simulink model "POParAgRL"  (R2015a)
settings: Solver=ode45  StartTime=0.0  StopTime=3  FixedStep=0.00001  RelTol=1e-5
settings Model: Creator=user  LastModifiedBy=user
settings SolverCC: ZeroCrossAlgorithm=Adaptive
settings DebuggingCC: UnderspecifiedInitializationDetection=Classic

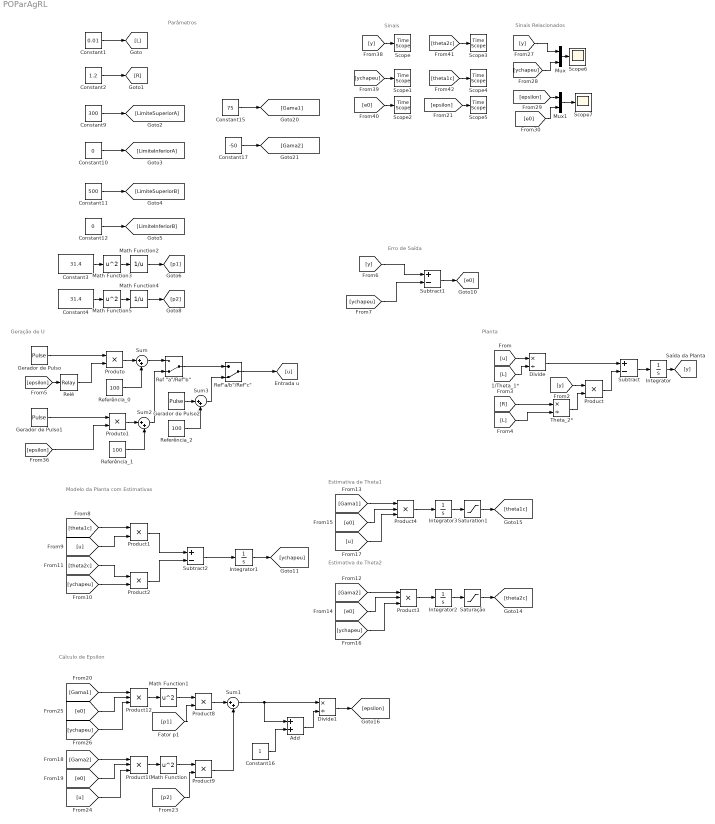
== system POParAgRL ==
  note: Modelo da Planta com Estimativas
  note: Sinais Relacionados
  note: Cálculo de Epsilon
  note: Estimativa de Theta1
  note: Estimativa de Theta2
  note: Geração de U
  note: Erro de Saída
  note: Parâmetros
  note: Sinais
  note: Planta
  Add : Sum  AccumDataTypeStr=double
  Constant1 : Constant  Value=0.01
  Constant10 : Constant  Value=0
  Constant11 : Constant  Value=500
  Constant12 : Constant  Value=0
  Constant15 : Constant  Value=75
  Constant16 : Constant
  Constant17 : Constant  Value=-50
  Constant2 : Constant  Value=1.2
  Constant3 : Constant  Value=31.4
  Constant4 : Constant  Value=31.4
  Constant9 : Constant  Value=300
  Divide : Product  Inputs=*/
  Divide1 : Product  Inputs=*/  OutDataTypeStr=double
  Gerador de Pulso : DiscretePulseGenerator  PulseType=Time based  Amplitude=100  Period=0.01  PulseWidth=50
  Gerador de Pulso1 : DiscretePulseGenerator  PulseType=Time based  Amplitude=100  Period=0.01  PulseWidth=50
  Gerador de Pulso2 : DiscretePulseGenerator  PulseType=Time based  Amplitude=100  Period=0.01  PulseWidth=50
  Integrator : Integrator
  Integrator1 : Integrator
  Integrator2 : Integrator  InitialCondition=70
  Integrator3 : Integrator  InitialCondition=80
  Math Function{,1,3,5} (4 alike) : Math  Operator=square  SaturateOnIntegerOverflow=on
  Math Function2 : Math  Operator=reciprocal  SaturateOnIntegerOverflow=on
  Math Function4 : Math  Operator=reciprocal  SaturateOnIntegerOverflow=on
  Mux : Mux  Inputs=2
  Mux1 : Mux  Inputs=2
  Product{,1..2,8..9} (5 alike) : Product
  Product{3..4,10,12} (4 alike) : Product  Inputs=3
  Produto : Product
  Produto1 : Product
  "Ref \"a\"/Ref\"b\"" : ManualSwitch  CurrentSetting=0
  "Ref\"a/b\"/Ref\"c\"" : ManualSwitch  CurrentSetting=0
  Referência_0 : Constant  Value=100
  Referência_1 : Constant  Value=100
  Referência_2 : Constant  Value=100
  Relé : Relay  OnSwitchValue=0.5  OffSwitchValue=0.5
  Saturation1 : Saturate  UpperLimit=300  LowerLimit=0
  Saturação : Saturate  UpperLimit=500  LowerLimit=0
  Scope{,1..5} (6 alike) : TimeScope
  Scope6 : Scope
      settings: YMin=79.1666  YMax=87.5  SaveName=ScopeData4
  Scope7 : Scope
      settings: YMin=-5e-08  YMax=6e-08  SaveName=ScopeData5
  Subtract : Sum  Inputs=+-
  Subtract1 : Sum  Inputs=+-
  Subtract2 : Sum  Inputs=+-
  Sum{,1..3} (4 alike) : Sum  Inputs=|++
  Theta_2* : Product  Inputs=*/
  wires:
  Referência_0/1 -> Sum/2
  [L] -> Divide/2
  Theta_2*/1 -> Product/2
  [L] -> Theta_2*/2
  [R] -> Theta_2*/1
  Product/1 -> Subtract/2
  Divide/1 -> Subtract/1
  Subtract/1 -> Integrator/1
  Integrator/1 -> [y]
  [y] -> Product/1
  Sum/1 -> "Ref \"a\"/Ref\"b\""/1
  [u] -> Divide/1
  [y] -> Subtract1/1
  [ychapeu] -> Subtract1/2
  Subtract1/1 -> [e0]
  Constant1/1 -> [L]
  Constant2/1 -> [R]
  Product1/1 -> Subtract2/1
  Subtract2/1 -> Integrator1/1
  Product2/1 -> Subtract2/2
  [u] -> Product1/2
  [theta1c] -> Product1/1
  Integrator1/1 -> [ychapeu]
  [e0] -> Product3/2
  [Gama2] -> Product3/1
  [Gama1] -> Product4/1
  [e0] -> Product4/2
  Product3/1 -> Integrator2/1
  Product4/1 -> Integrator3/1
  Integrator3/1 -> Saturation1/1
  Integrator2/1 -> Saturação/1
  Produto/1 -> Sum/1
  Gerador de Pulso/1 -> Produto/1
  Product10/1 -> Math Function/1
  Product12/1 -> Math Function1/1
  Math Function1/1 -> Product8/1
  Math Function/1 -> Product9/1
  [p1] -> Product8/2
  [p2] -> Product9/2
  Product9/1 -> Sum1/2
  Product8/1 -> Sum1/1
  Constant9/1 -> [LimiteSuperiorA]
  Constant10/1 -> [LimiteInferiorA]
  Constant11/1 -> [LimiteSuperiorB]
  Constant12/1 -> [LimiteInferiorB]
  Math Function2/1 -> [p1]
  [y] -> Scope/1
  [ychapeu] -> Scope1/1
  [e0] -> Scope2/1
  [theta2c] -> Scope3/1
  [theta1c] -> Scope4/1
  Constant17/1 -> [Gama2]
  Constant15/1 -> [Gama1]
  Divide1/1 -> [epsilon]
  Add/1 -> Divide1/2
  Constant16/1 -> Add/2
  Sum1/1 -> Add/1, Divide1/1
  [epsilon] -> Relé/1
  Saturação/1 -> [theta2c]
  Saturation1/1 -> [theta1c]
  [Gama2] -> Product10/1
  [u] -> Product10/3
  [e0] -> Product12/2
  [Gama1] -> Product12/1
  [ychapeu] -> Product12/3
  Relé/1 -> Produto/2
  [epsilon] -> Scope5/1
  [ychapeu] -> Mux/2
  [y] -> Mux/1
  Mux/1 -> Scope6/1
  [epsilon] -> Mux1/1
  [e0] -> Mux1/2
  Mux1/1 -> Scope7/1
  Math Function3/1 -> Math Function2/1
  Constant3/1 -> Math Function3/1
  Math Function5/1 -> Math Function4/1
  Constant4/1 -> Math Function5/1
  Math Function4/1 -> [p2]
  "Ref \"a\"/Ref\"b\""/1 -> "Ref\"a/b\"/Ref\"c\""/1
  Referência_1/1 -> Sum2/2
  Produto1/1 -> Sum2/1
  Gerador de Pulso1/1 -> Produto1/1
  [epsilon] -> Produto1/2
  Sum2/1 -> "Ref \"a\"/Ref\"b\""/2
  [theta2c] -> Product2/1
  [ychapeu] -> Product2/2
  [ychapeu] -> Product3/3
  [u] -> Product4/3
  [e0] -> Product10/2
  "Ref\"a/b\"/Ref\"c\""/1 -> [u]
  Sum3/1 -> "Ref\"a/b\"/Ref\"c\""/2
  Gerador de Pulso2/1 -> Sum3/1
  Referência_2/1 -> Sum3/2
